simulink model "Controller_Algorithm"  (R2018a)
settings: Solver=FixedStepAuto  StartTime=0.0  StopTime=inf  RelTol=1e-3  EnableMultiTasking=on
undefined symbols (not defined in the file): DiscIntNeverNeededParam, Fc, Kd, Ki, Kp, Ts
settings Model: ExtModeTrigDuration=2  Creator=pmaier  LastModifiedBy=scastro
settings OptimizationCC: EnhancedBackFolding=on  PassReuseOutputArgsAs=Individual arguments  MaxStackSize=64  OptimizeBlockOrder=speed  DifferentSizesBufferReuse=on  OptimizationCustomize=off
settings DebuggingCC: ParameterTunabilityLossMsg=error
settings HardwareCC: ProdBitPerInt=16  ProdBitPerPointer=16  ProdBitPerSizeT=16  ProdBitPerPtrDiffT=16  ProdLargestAtomicFloat=None  ProdWordSize=8  ProdHWDeviceType=Atmel->AVR
settings SFSimCC: MATLABDynamicMemAlloc=off
settings RTWCC: SystemTargetFile=ert.tlc  HardwareBoard=Arduino Uno  TLCOptions=-aInlineSetEventsForThisBaseRateFcn=TLC_FALSE -aSuppressMultiTaskScheduler=TLC_FALSE -aRateBasedStepFcn=1  TemplateMakefile=ert_default_tmf  GenerateReport=on  Toolchain=Arduino AVR  BuildConfiguration=Faster Runs  IncludeHyperlinkInReport=on  LaunchReport=on  GenerateTraceInfo=on  GenerateTraceReport=on  GenerateTraceReportSl=on  GenerateTraceReportSf=on  GenerateTraceReportEml=on
settings CodeAppCC: ForceParamTrailComments=on  IgnoreCustomStorageClasses=off  OperatorAnnotations=on  SimulinkDataObjDesc=on  SFDataObjDesc=on  InsertBlockDesc=on
settings ERTTargetCC: SupportContinuousTime=on  SupportVariableSizeSignals=on

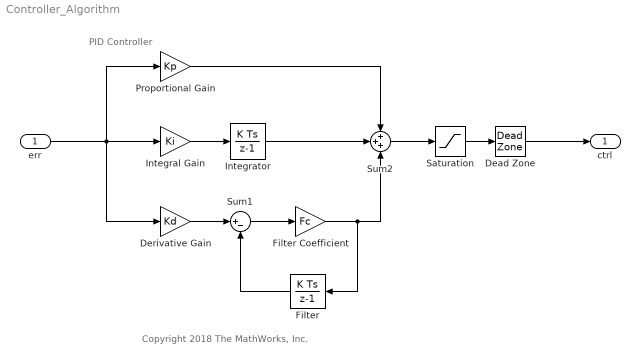
== system Controller_Algorithm ==
  note: Copyright 2018 The MathWorks, Inc.
  note: PID Controller
  err : Inport  OutDataTypeStr=double  PortDimensions=[1 1]  SampleTime=[0.01,0]
  Dead Zone : DeadZone  LowerValue=-0.2  UpperValue=0.2  SaturateOnIntegerOverflow=on
  Derivative Gain : Gain  Gain=Kd
  Filter : DiscreteIntegrator  DisableCoverage=on  SampleTime=Ts  ICPrevOutput=DiscIntNeverNeededParam  ICPrevScaledInput=DiscIntNeverNeededParam
  Filter Coefficient : Gain  Gain=Fc
  Integral Gain : Gain  Gain=Ki
  Integrator : DiscreteIntegrator  SampleTime=Ts  ICPrevOutput=DiscIntNeverNeededParam  ICPrevScaledInput=DiscIntNeverNeededParam
  Proportional Gain : Gain  Gain=Kp
  Saturation : Saturate  UpperLimit=8  LowerLimit=-8
  Sum1 : Sum  Inputs=|+-
  Sum2 : Sum  Inputs=+++
  ctrl : Outport  OutDataTypeStr=double  PortDimensions=1  SampleTime=[0.01,0]
  wires:
  Saturation/1 -> Dead Zone/1
  Sum1/1 -> Filter Coefficient/1
  Filter/1 -> Sum1/2
  Integrator/1 -> Sum2/2
  Proportional Gain/1 -> Sum2/1
  Filter Coefficient/1 -> Filter/1, Sum2/3
  err/1 -> Integral Gain/1, Proportional Gain/1, Derivative Gain/1
  Integral Gain/1 -> Integrator/1
  Derivative Gain/1 -> Sum1/1
  Sum2/1 -> Saturation/1
  Dead Zone/1 -> ctrl/1
